simulink model "LatSim"  (R2020a)
settings: Solver=VariableStepAuto  StartTime=0.0  StopTime=300  FixedStep=0.01  RelTol=1e-3
values from neighbouring files (symbols this model uses):
  ALateralFull = ALateralFull-BLateralFull*kFull    [Lateral.m]
  BLateralFull = [YCA YCR;LCA LCR;NCA NCR; 0 0; 0 0]    [Lateral.m]
  CLateralFull = eye(5)    [Lateral.m]
  DLateralFull = zeros(5,2)    [Lateral.m]
undefined symbols (not defined in the file or in its folder): g, sigbuilder_block
libraries: cstblocks x3, simulink_extras x3, simulink x1
settings Model: Creator=moham  LastModifiedBy=MuAyman

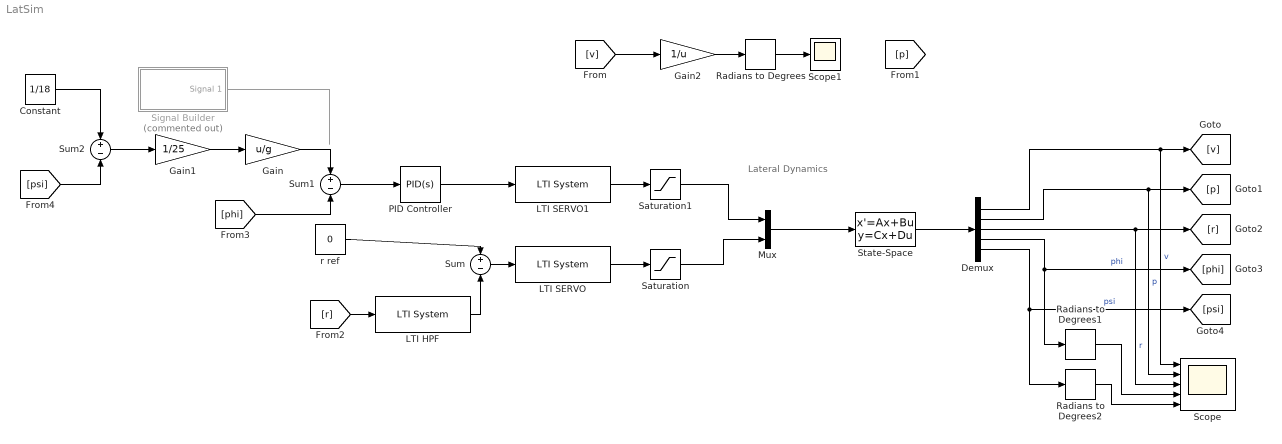
== system LatSim ==
  note: Lateral Dynamics
  Constant : Constant  Value=1/18
  Demux : Demux  Outputs=5
  Gain : Gain  Gain=u/g
  Gain1 : Gain  Gain=1/25
  Gain2 : Gain  Gain=1/u
  LTI HPF : cstblocks/LTI System  sys=tf(0.1,[0.1 1])  IC=[]
  LTI SERVO : cstblocks/LTI System  sys=-tf(10,[1 10])  IC=[]
  LTI SERVO1 : cstblocks/LTI System  sys=tf(10,[1 10])  IC=[]
  Mux : Mux  Inputs=2
  PID Controller : simulink/Continuous/PID Controller  Controller=PID  Form=Parallel  TimeDomain=Continuous-time  UseExternalTs=off  SampleTime=-1  IntegratorMethod=Forward Euler  FilterMethod=Forward Euler  ControllerParametersSource=internal  P=4.21258744913478  I=0.102825649265939  D=15.0785551628416  UseFilter=on  N=352.938314261655  TunerSelectOption=Transfer Function Based (PID Tuner App)  InitialConditionSource=internal  InitialConditionForIntegrator=0  InitialConditionForFilter=0  DifferentiatorICPrevScaledInput=0  ExternalReset=none  TrackingMode=off  Kt=1  LimitOutput=off  UpperSaturationLimit=inf  LowerSaturationLimit=-inf  LinearizeAsGain=on  AntiWindupMode=none  Kb=1  POutMin=[]  POutMax=[]  IOutMin=[]  IOutMax=[]  DOutMin=[]  DOutMax=[]  NOutMin=[]  NOutMax=[]  SumOutMin=[]  SumOutMax=[]  SaturationOutMin=[]  SaturationOutMax=[]  PParamMin=[]  PParamMax=[]  IParamMin=[]  IParamMax=[]  DParamMin=[]  DParamMax=[]  NParamMin=[]  NParamMax=[]  KbParamMin=[]  KbParamMax=[]  KtParamMin=[]  KtParamMax=[]  KbOutMin=[]  KbOutMax=[]  KtOutMin=[]  KtOutMax=[]  IntegratorOutMin=[]  IntegratorOutMax=[]  FilterOutMin=[]  FilterOutMax=[]  SumI1OutMin=[]  SumI1OutMax=[]  SumI2OutMin=[]  SumI2OutMax=[]  SumI3OutMin=[]  SumI3OutMax=[]  SumI4OutMin=[]  SumI4OutMax=[]  SumDOutMin=[]  SumDOutMax=[]  DifferentiatorOutMin=[]  DifferentiatorOutMax=[]  FilterDiffOutCoefMin=[]  FilterDiffOutCoefMax=[]  ReciprocalOutMin=[]  ReciprocalOutMax=[]  SumDenOutMin=[]  SumDenOutMax=[]  SumNumOutMin=[]  SumNumOutMax=[]  DivideOutMin=[]  DivideOutMax=[]  UdiffTsProdOutMin=[]  UdiffTsProdOutMax=[]  NTsProdOutMin=[]  NTsProdOutMax=[]  UintegralTsProdOutMin=[]  UintegralTsProdOutMax=[]  UngainTsProdOutMin=[]  UngainTsProdOutMax=[]  IntegratorContinuousStateAttributes=''  IntegratorStateMustResolveToSignalObject=off  IntegratorRTWStateStorageClass=Auto  FilterContinuousStateAttributes=''  FilterStateMustResolveToSignalObject=off  FilterRTWStateStorageClass=Auto  ParallelPVariant=InternalParameters  IdealPVariant=Disabled  IVariant=InternalParameters  DVariant=InternalParameters  IntegratorVariant=Continuous  SatVariant=Disabled  AWVariant=Passthrough  PCopyVariant=Disabled  TRVariant=Disabled  FdbkBlocksVariant=Forward  IdealPFdbkVariant=Disabled  SatFdbkVariant=Disabled  DerivativeFilterVariant=ContFilter  NVariant=InternalParameters  NCopyVariant=Disabled  FilterICVariant=InternalICsFilter  IntegratorICVariant=InternalICs  ExternalResetVariant=Disabled  TRSumVariant=Passthrough  SumFdbkVariant=Disabled  SumVariant=Sum_PID  TsampFilterVariant=InternalTs  TsampNgainVariant=Passthrough  TsampIntegralVariant=Passthrough
  Radians to Degrees : simulink_extras/Transformations/Radians to Degrees
  Radians to Degrees1 : simulink_extras/Transformations/Radians to Degrees
  Radians to Degrees2 : simulink_extras/Transformations/Radians to Degrees
  Saturation : Saturate
  Saturation1 : Saturate
  Scope : Scope  NumInputPorts=5
  Scope1 : Scope
  Signal Builder : Subsystem  Tag=STV Subsys  Commented=on  LoadFcn=sigbuilder_block('load');  StartFcn=sigbuilder_block('start');  StopFcn=sigbuilder_block('stop');  ClipboardFcn=sigbuilder_block('clipboard');  mask(Sigbuilder block){tuvar=[0:10]}
      mask help: Simulink:masks:SigbuilderBlock_MD
      mask init:
      | if ~strcmp(get_param(bdroot(gcbh),'SimulationStatus'),'stopped') tuvar = sigbuilder_block('maskInit'); end
      settings: CopyFcn=sigbuilder_block('copy');  DeleteFcn=sigbuilder_block('delete');  ModelCloseFcn=sigbuilder_block('modelClose');  PreSaveFcn=sigbuilder_block('preSave');  PauseFcn=sigbuilder_block('pause');  ContinueFcn=sigbuilder_block('continue');  NameChangeFcn=sigbuilder_block('namechange');  OpenFcn=sigbuilder_block('open',[195.75 104.25 550.5 359.25 ]);  CloseFcn=sigbuilder_block('close');
      mask Display: plot(0, 0, 100, 100,[2, 2, 32, 32, 2], [68, 8, 8, 68, 68],[32, 2], [38, 38], [32, 19, 2],[53, 60, 44], [32, 17, 17, 2],[16, 16, 31, 31]);txt = getActiveGroup(gcbh);text(2, 100, txt,'verticalAlignment', 'top');
  State-Space : StateSpace  A=ALateralFull  B=BLateralFull  C=CLateralFull  D=DLateralFull  InitialCondition=0
  Sum : Sum  Inputs=+-
  Sum1 : Sum  Inputs=+-
  Sum2 : Sum  Inputs=+-
  r ref : Constant  Value=0
  wires:
  Demux/1 -> Scope/1, [v]  "v"
  State-Space/1 -> Demux/1
  Demux/2 -> Scope/2, [p]  "p"
  Mux/1 -> State-Space/1
  Saturation/1 -> Mux/2
  Demux/3 -> Scope/3, [r]  "r"
  Demux/4 -> Radians to Degrees1/1, [phi]  "phi"
  Demux/5 -> Radians to Degrees2/1, [psi]  "psi"
  [r] -> LTI HPF/1
  LTI SERVO/1 -> Saturation/1
  Sum/1 -> LTI SERVO/1
  LTI HPF/1 -> Sum/2
  r ref/1 -> Sum/1
  Saturation1/1 -> Mux/1
  LTI SERVO1/1 -> Saturation1/1
  [phi] -> Sum1/2
  PID Controller/1 -> LTI SERVO1/1
  Sum1/1 -> PID Controller/1
  [psi] -> Sum2/2
  Constant/1 -> Sum2/1
  Sum2/1 -> Gain1/1
  Gain1/1 -> Gain/1
  Gain/1 -> Sum1/1
  [v] -> Gain2/1
  Signal Builder/1(Signal 1) -> ?
  Gain2/1 -> Radians to Degrees/1
  Radians to Degrees/1 -> Scope1/1
  Radians to Degrees1/1 -> Scope/4
  Radians to Degrees2/1 -> Scope/5

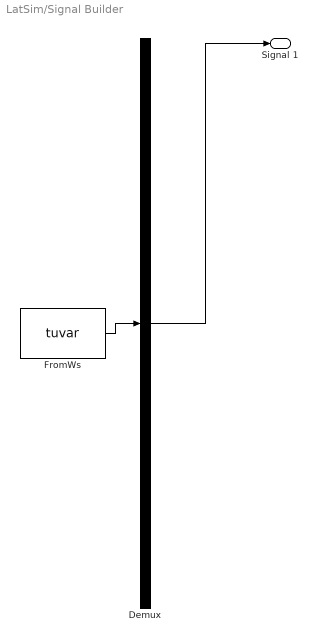
== system LatSim/Signal Builder ==
  Demux : Demux  Tag=STV Demux  Outputs=1
      settings: DisplayOption=none
  FromWs : FromWorkspace  Tag=STV FromWs  VariableName=tuvar
      SigBuilderData=|
      | common.afterFinalStr = 'Extrapolate'
      | common.sampleTime = 0
      | dataSet.timeRange = [0 200]
      | dataSet.name = 'Group 1'
      | sbobj.Groups.Name = 'Group 1'
      | sbobj.Groups.Signals.Name = 'Signal 1'
      | sbobj.Groups.Signals.XData = [0 3 3 20 20 200]
      | sbobj.Groups.Signals.YData = [0 0 30 30 0 0]
      | sbobj.Groups.TimeRange = [0 200]
  Signal 1 : Outport  Tag=STV Outport
  wires:
  Demux/1 -> Signal 1/1
  FromWs/1 -> Demux/1
